simulink model "dev_RigTest_networkOnly_withPredictor"  (R2020b)
settings: Solver=VariableStepAuto  StartTime=0.0  StopTime=1500  RelTol=1e-3
libraries: IMT_Library x4, simulink_extras x4, slpidlib x1
settings Model: Creator=Mr_Li  LastModifiedBy=Mr_Li

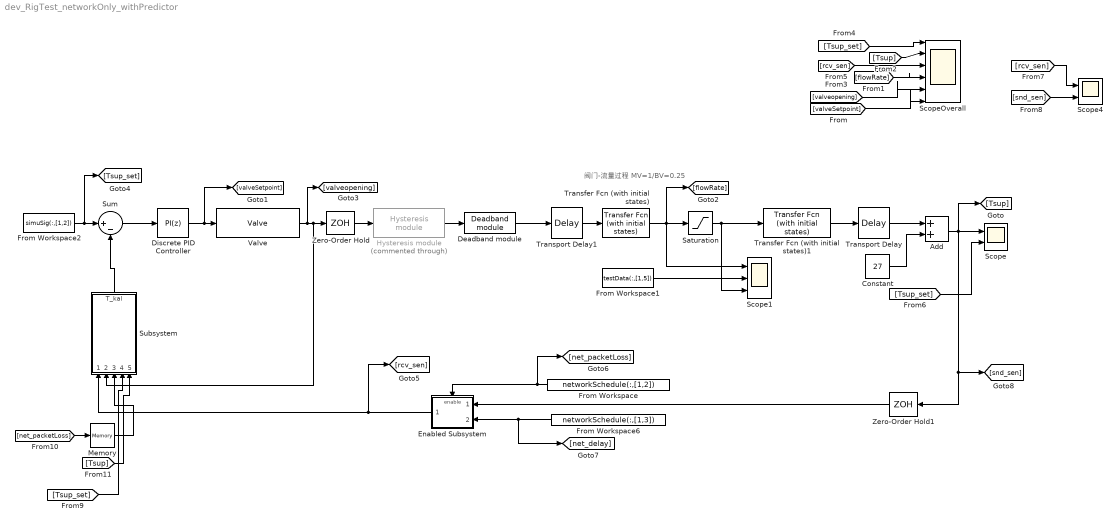
== system dev_RigTest_networkOnly_withPredictor ==
  note: 阀门-流量过程
      | MV=1/BV=0.25
  Add : Sum
  Constant : Constant  Value=27
  Deadband module : IMT_Library/Deadband module  upper=22.5  lower=6.5
      settings: SourceProductName=Imitation
  Discrete PID Controller : slpidlib/PID Controller  Controller=PI  Form=Parallel  TimeDomain=Discrete-time  UseExternalTs=off  SampleTime=1  IntegratorMethod=Forward Euler  FilterMethod=Forward Euler  ControllerParametersSource=internal  P=0.5  I=0.00715  D=0  UseFilter=on  N=100  TunerSelectOption=Frequency Response Based  InitialConditionSource=internal  InitialConditionForIntegrator=0  InitialConditionForFilter=0  DifferentiatorICPrevScaledInput=0  ExternalReset=none  TrackingMode=off  Kt=1  LimitOutput=off  SatLimitsSource=internal  UpperSaturationLimit=inf  LowerSaturationLimit=-inf  LinearizeAsGain=off  AntiWindupMode=none  Kb=1  POutMin=[]  POutMax=[]  IOutMin=[]  IOutMax=[]  DOutMin=[]  DOutMax=[]  NOutMin=[]  NOutMax=[]  SumOutMin=[]  SumOutMax=[]  SaturationOutMin=[]  SaturationOutMax=[]  PParamMin=[]  PParamMax=[]  IParamMin=[]  IParamMax=[]  DParamMin=[]  DParamMax=[]  NParamMin=[]  NParamMax=[]  KbParamMin=[]  KbParamMax=[]  KtParamMin=[]  KtParamMax=[]  KbOutMin=[]  KbOutMax=[]  KtOutMin=[]  KtOutMax=[]  IntegratorOutMin=[]  IntegratorOutMax=[]  FilterOutMin=[]  FilterOutMax=[]  SumI1OutMin=[]  SumI1OutMax=[]  SumI2OutMin=[]  SumI2OutMax=[]  SumI3OutMin=[]  SumI3OutMax=[]  SumI4OutMin=[]  SumI4OutMax=[]  SumDOutMin=[]  SumDOutMax=[]  DifferentiatorOutMin=[]  DifferentiatorOutMax=[]  FilterDiffOutCoefMin=[]  FilterDiffOutCoefMax=[]  ReciprocalOutMin=[]  ReciprocalOutMax=[]  SumDenOutMin=[]  SumDenOutMax=[]  SumNumOutMin=[]  SumNumOutMax=[]  DivideOutMin=[]  DivideOutMax=[]  UdiffTsProdOutMin=[]  UdiffTsProdOutMax=[]  NTsProdOutMin=[]  NTsProdOutMax=[]  UintegralTsProdOutMin=[]  UintegralTsProdOutMax=[]  UngainTsProdOutMin=[]  UngainTsProdOutMax=[]  IntegratorContinuousStateAttributes=''  IntegratorStateMustResolveToSignalObject=off  IntegratorRTWStateStorageClass=Auto  FilterContinuousStateAttributes=''  FilterStateMustResolveToSignalObject=off  FilterRTWStateStorageClass=Auto  ParallelPVariant=InternalParameters  IdealPVariant=Disabled  IVariant=InternalParameters  DVariant=Disabled  IntegratorVariant=Discrete  SatVariant=Disabled  AWVariant=Passthrough  PCopyVariant=Disabled  TRVariant=Disabled  FdbkBlocksVariant=Forward  IdealPFdbkVariant=Disabled  SatFdbkVariant=Disabled  DerivativeFilterVariant=Disabled  NVariant=Disabled  NCopyVariant=Disabled_SignalSpec  FilterICVariant=Disabled  IntegratorICVariant=InternalICs  ExternalResetVariant=Disabled  TRSumVariant=Passthrough  SumFdbkVariant=Disabled  SumVariant=Sum_PI  TsampFilterVariant=InternalTs  TsampNgainVariant=Passthrough  TsampIntegralVariant=Passthrough  ExternalSaturationOutDataTypeStr=Inherit: Same as second input
  Enabled Subsystem : Subsystem  TreatAsAtomicUnit=on
  From Workspace : FromWorkspace  VariableName=networkSchedule(:,[1,2])  SampleTime=1
  From Workspace1 : FromWorkspace  VariableName=testData(:,[1,5])
  From Workspace2 : FromWorkspace  VariableName=simuSig(:,[1,2])  SampleTime=1
  From Workspace6 : FromWorkspace  VariableName=networkSchedule(:,[1,3])  OutDataTypeStr=double  SampleTime=0.001  OutputAfterFinalValue=Holding final value
  Hysteresis module : IMT_Library/Hysteresis module  Commented=through  hysteresisSize=4.5
      settings: SourceProductName=Imitation
  Memory : Memory  InheritSampleTime=on
  Saturation : Saturate  UpperLimit=0.25  LowerLimit=0
  Scope : Scope  NumInputPorts=2
  Scope1 : Scope  NumInputPorts=3
  Scope4 : Scope  NumInputPorts=2
  ScopeOverall : Scope  NumInputPorts=6
  Subsystem : Subsystem
  Sum : Sum  Inputs=|+-
  Transfer Fcn (with initial states) : simulink_extras/Additional Linear/Transfer Fcn (with initial states)  N=[0.032]  D=[3.6 1]  X0=0
  Transfer Fcn (with initial states)1 : simulink_extras/Additional Linear/Transfer Fcn (with initial states)  N=[105]  D=[380 40 1]  X0=0
  Transport Delay : TransportDelay  DelayTime=0
  Transport Delay1 : TransportDelay  DelayTime=3
  Valve : IMT_Library/Valve  upper=101  lower=1.2  movementThreshold=1
      settings: SourceProductName=Imitation
  Zero-Order Hold : ZeroOrderHold
  Zero-Order Hold1 : ZeroOrderHold
  wires:
  Hysteresis module/1 -> Deadband module/1
  Constant/1 -> Add/2
  Transport Delay1/1 -> Transfer Fcn (with initial states)/1
  Valve/1 -> Subsystem/2(Current Valve), Zero-Order Hold/1, [valveopening]
  Transfer Fcn (with initial states)/1 -> Saturation/1, [flowRate], Scope1/1
  Discrete PID Controller/1 -> Valve/1, [valveSetpoint]
  Sum/1 -> Discrete PID Controller/1
  From Workspace1/1 -> Scope1/2
  Saturation/1 -> Scope1/3, Transfer Fcn (with initial states)1/1
  Deadband module/1 -> Transport Delay1/1
  Zero-Order Hold/1 -> Hysteresis module/1
  Transport Delay/1 -> Add/1
  Transfer Fcn (with initial states)1/1 -> Transport Delay/1
  From Workspace6/1 -> [net_delay], Enabled Subsystem/2(delay)
  Add/1 -> Zero-Order Hold1/1, [snd_sen], Scope/1, [Tsup]
  From Workspace/1 -> [net_packetLoss], Enabled Subsystem/Enable
  [Tsup_set] -> Scope/2
  From Workspace2/1 -> [Tsup_set], Sum/1
  [Tsup_set] -> ScopeOverall/1
  [Tsup] -> ScopeOverall/2
  [rcv_sen] -> ScopeOverall/3
  [flowRate] -> ScopeOverall/4
  [valveopening] -> ScopeOverall/5
  [valveSetpoint] -> ScopeOverall/6
  Zero-Order Hold1/1 -> Enabled Subsystem/1(data)
  [snd_sen] -> Scope4/2
  [rcv_sen] -> Scope4/1
  Enabled Subsystem/1(Out1) -> [rcv_sen], Subsystem/1(T_rcv)
  [net_packetLoss] -> Memory/1
  Subsystem/1(T_kal) -> Sum/2
  Memory/1 -> Subsystem/3(isRcv)
  [Tsup] -> Subsystem/5(Tsup)
  [Tsup_set] -> Subsystem/4(Tsup,set)

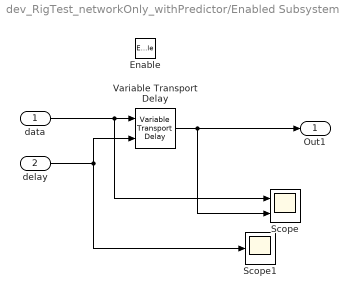
== system dev_RigTest_networkOnly_withPredictor/Enabled Subsystem ==
  data : Inport
  delay : Inport  Port=2
  Enable : EnablePort
  Scope : Scope  NumInputPorts=2
  Scope1 : Scope
  Variable Transport Delay : VariableTransportDelay  MaximumDelay=10  MaximumPoints=4000  ZeroDelay=on
  Out1 : Outport
  wires:
  data/1 -> Variable Transport Delay/1, Scope/1
  delay/1 -> Variable Transport Delay/2, Scope1/1
  Variable Transport Delay/1 -> Out1/1, Scope/2

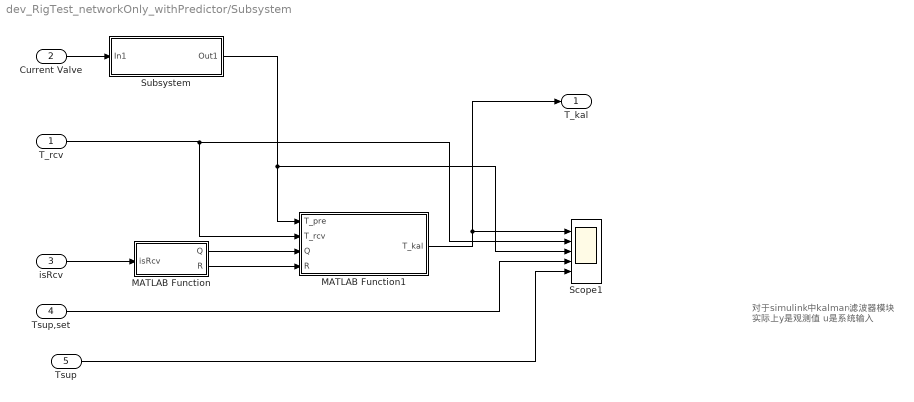
== system dev_RigTest_networkOnly_withPredictor/Subsystem ==
  note: 对于simulink中kalman滤波器模块
      | 实际上y是观测值
      | u是系统输入
  T_rcv : Inport
  Current Valve : Inport  Port=2
  isRcv : Inport  Port=3
  Tsup,set : Inport  Port=4
  Tsup : Inport  Port=5
  MATLAB Function : MATLAB Function  TreatAsAtomicUnit=on
  MATLAB Function1 : MATLAB Function  TreatAsAtomicUnit=on
  Scope1 : Scope  NumInputPorts=5
  Subsystem : Subsystem
  T_kal : Outport
  wires:
  T_rcv/1 -> MATLAB Function1/2(T_rcv), Scope1/2
  isRcv/1 -> MATLAB Function/1(isRcv)
  MATLAB Function/1(Q) -> MATLAB Function1/3(Q)
  MATLAB Function/2(R) -> MATLAB Function1/4(R)
  MATLAB Function1/1(T_kal) -> T_kal/1, Scope1/1
  Subsystem/1(Out1) -> Scope1/3, MATLAB Function1/1(T_pre)
  Current Valve/1 -> Subsystem/1(In1)
  Tsup,set/1 -> Scope1/4
  Tsup/1 -> Scope1/5

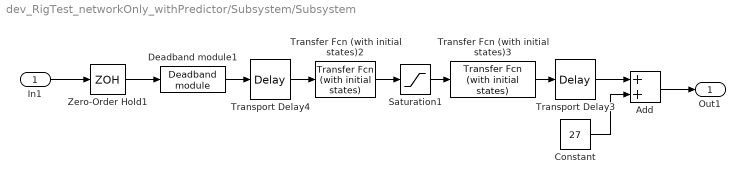
== system dev_RigTest_networkOnly_withPredictor/Subsystem/Subsystem ==
  In1 : Inport
  Add : Sum
  Constant : Constant  Value=27
  Deadband module1 : IMT_Library/Deadband module  upper=22.5  lower=6.5
      settings: SourceProductName=Imitation
  Saturation1 : Saturate  UpperLimit=0.25  LowerLimit=0
  Transfer Fcn (with initial states)2 : simulink_extras/Additional Linear/Transfer Fcn (with initial states)  N=[0.032]  D=[3.6 1]  X0=0
  Transfer Fcn (with initial states)3 : simulink_extras/Additional Linear/Transfer Fcn (with initial states)  N=[105]  D=[380 40 1]  X0=0
  Transport Delay3 : TransportDelay  DelayTime=0
  Transport Delay4 : TransportDelay  DelayTime=3
  Zero-Order Hold1 : ZeroOrderHold
  Out1 : Outport
  wires:
  Add/1 -> Out1/1
  Transport Delay3/1 -> Add/1
  Zero-Order Hold1/1 -> Deadband module1/1
  Saturation1/1 -> Transfer Fcn (with initial states)3/1
  Deadband module1/1 -> Transport Delay4/1
  Transfer Fcn (with initial states)3/1 -> Transport Delay3/1
  In1/1 -> Zero-Order Hold1/1
  Transfer Fcn (with initial states)2/1 -> Saturation1/1
  Constant/1 -> Add/2
  Transport Delay4/1 -> Transfer Fcn (with initial states)2/1

== matlab function dev_RigTest_networkOnly_withPredictor/Subsystem/MATLAB Function ==
  data: isRcv input; Q output; R output
function [Q,R] = fcn(isRcv)
% function [Q,R,lsCount] = fcn(isRcv)
persistent lossCount;

if(isempty(lossCount))
    lossCount=0;
end

if(isRcv==0)
%     丢包
    lossCount=lossCount+1;
%     Q=0.05;
%     R=0.36;
    Q=0.05-0.0005*lossCount;
    R=0.36+0.0005*lossCount;
%     Q=0.01/lossCount;%0.05/lossCount;
    if(Q<0)
        Q=0;%0.36;
    end
    if(R>1)
        R=1;
    end
    

else
%     接收正常
    lossCount=0; %重置计数器
    Q=0.98;
    R=0.01;
end
% lsCount=lossCount;
end

== matlab function dev_RigTest_networkOnly_withPredictor/Subsystem/MATLAB Function1 ==
  settings: updateMethod=DISCRETE  sampleTime=1
  data: T_pre input; T_kal output; T_rcv input; Q input; R input
function T_kal  = fcn(T_pre,T_rcv,Q,R)
persistent P_previous;
if(isempty(P_previous))
    P_previous=1;
end
    P_pre=P_previous+Q;
    K=P_pre/(P_pre+R);%K(k)???????
    T_kal=T_pre+K*(T_rcv-T_pre);
    P_kal=P_pre-(K*P_pre);
    P_previous=P_kal;
end
